simulink library "IOBlock_Library_TTC580"  (R2021a)
settings: Solver=ode45  StartTime=0.0  StopTime=10.0  RelTol=1e-3
PreLoadFcn:
  | addpath(genpath(fileparts(which('IOBlock_Library_TTC580'))));
  | %addpath(genpath(fileparts(which('IOBlock_Library_TTC580.mdl'))))
  | try
  | addpath(genpath([fileparts(which('IOBlock_Library_TTC580')),'\..\DBC_Importer']));
  | addpath(genpath([fileparts(which('IOBlock_Library_TTC580')),'\..\EEPROM_Importer']));
  | addpath(genpath([fileparts(which('IOBlock_Library_TTC580')),'\..\UserDoc']));
  | catch
  | warning('IOBlock_Library_TTC580: add path to DBC_Importer and EEPROM_Importer manually');
  | end
  | try
  | if exist('..\CustomPackage\scripts\OpenAllPackages.m','file')
  |      run('..\CustomPackage\scripts\OpenAllPackages.m'); %always available, ggf. empty
  | end
  | catch
  | warning('A problem occurred opening automatically the CustomPackage. Please open libraries manually');
  | end
  | try
  | set_param(0,'EditorSmartEditingHotParam','off');
  | catch
  | warning('Simlink preferences for ''Edit key parameter when adding new blocks'' needs to be unchecked manually');
  | end
undefined symbols (not defined in the file or in its folder): ADC_Absolute_10V, ADC_Absolute_32V, ADC_Absolute_5V, ADC_BoardTemp, ADC_ChannelInit, ADC_Current, ADC_Get, ADC_K15_, ADC_Ratiometric_10V, ADC_Ratiometric_5V, ADC_Resistive, ADC_SensorSupply, ADC_UBAT, bit_packing, bit_unpacking, CAN_ConfigMsg, compare2error, compare2FET_PROT_REENABLE, crc32_calc_intern, CRC32_EEPROM_Read, CRC32_EEPROM_Write, DIAG_EnterSafestate, DIAG_Status, DIAG_Status_internal, EEPROM_Mirror, EEPROM_Read, EEPROM_Read_OffsetIn, EEPROM_Read_Raw, EEPROM_Write, EEPROM_Write_OffsetIn, EEPROM_Write_Raw, EnterSafestate, FPU_Handler, Get_DI, Get_DI_VarThreshold, Get_K15_, Get_Pulse_Freq_Curr, Get_Pulse_Freq_Volt, Get_WakeUp, GetDateAndTime, IO_ADC_ResetProtection, IO_Blk_Lib_TTC500, IO_CAN_ReadMsg, IO_CAN_WriteMsg, IO_DI_Get, IO_DI_Init, IO_DI_Init_Var, IO_DO_GetCur, IO_DO_GetVoltage, IO_DO_Init, IO_DO_ResetProtection, IO_DO_Set, IO_Driver_GetSerialNumber, IO_Driver_GetVersionOfDriver, IO_Driver_GetVersionOfFPGA, IO_EEPROM_GetStatus, IO_EEPROM_Init, IO_EEPROM_Read_raw, IO_EEPROM_Write, IO_EEPROM_Write_OffsetIn ... (+73)
libraries: simulink x43
(part 14 of 18)

== system IOBlock_Library_TTC580/PWM Blocks TTC580 IOlib/Set_PWM_Simple ==
  duty_cycle : Inport  OutDataTypeStr=uint16  PortDimensions=1
  IO_PWM_Init : Subsystem  LoadFcn=|  mask(IO_PWM_Init_Code){SampleTime=-1, ttlib=IO_Blk_Lib_TTC500, ttDescription=IO_PWM_Init, tt_iolib_version=0.19, pwm_channel=pwm_channel, frequency=frequency, polarity=num2str(polarity_high), diag_margin=num2str(diag_margin), safety_conf=NULL}
      | try
      | %
      | %Upgrade Information - standard BEGIN
      | new_color = 'blue';
      | new_ver = '0.19';
      | act_ver = get_param(gcb,'tt_iolib_version');
      | if not(strcmp(act_ver,new_ver))
      |     disp(['Upgrade block: ',gcb,char(10),'       Version: ',act_ver,' -> ',new_ver]);
      |     %switch - case for specific upgrade information e.g. additional parameter required 
      |     %Change appearance and version information
      |     set_param(gcb,'ForegroundColor',new_color);
      |     set_param(gcb,'tt_iolib_version',new_ver);
      | end
      | %Upgrade Information - standard END
      | catch
      | %Standard catch section BEGIN 
      | disp(' ');
      | disp('------------------------------------------------------------');
      | disp('An error occurred in a callback of the TTC580-BlockLib.');
      | disp(['Please check the parameters in the mask of ',gcb]);
      | disp('If you do not encounter any violations, then please '); 
      | disp('copy the following lines and report this to support@ttcontrol.com ');
      | disp('<< begin of error message dump >>');
      | disp(['Version of TTC580-BlockLib: ', get_param(gcb,'tt_iolib_version')]);
      | disp(get_param(gcb,'ttDescription'));
      | disp(gcb);
      | x=lasterror;disp(x.message);
      | disp(get_param(gcb,'MaskValues'));
      | disp(version);
      | disp(computer);
      | disp('<< end of error message dump >>');
      | disp('------------------------------------------------------------');
      | disp(' ');
      | %Standard catch section END
      | end
      mask help: Setup single PWM output.
      mask init:
      | %
      settings: CopyFcn=%deleted
      mask Help: web(which('IO_PWM.h'))
      mask Callback pwm_channel: %
      mask Callback frequency: %
      mask Callback polarity: %
      mask Callback diag_margin: %
      mask Callback safety_conf: %
  IO_PWM_ResetProtection : Subsystem  LoadFcn=|  mask(IO_PWM_ResetProtection_Code){SampleTime=-1, ttlib=IO_Blk_Lib_TTC500, ttDescription=IO_PWM_ResetProtection, tt_iolib_version=0.19, pwm_channel=pwm_channel}
      | try
      | %
      | %Upgrade Information - standard BEGIN
      | new_color = 'blue';
      | new_ver = '0.19';
      | act_ver = get_param(gcb,'tt_iolib_version');
      | if not(strcmp(act_ver,new_ver))
      |     disp(['Upgrade block: ',gcb,char(10),'       Version: ',act_ver,' -> ',new_ver]);
      |     %switch - case for specific upgrade information e.g. additional parameter required 
      |     %Change appearance and version information
      |     set_param(gcb,'ForegroundColor',new_color);
      |     set_param(gcb,'tt_iolib_version',new_ver);
      | end
      | %Upgrade Information - standard END
      | catch
      | %Standard catch section BEGIN 
      | disp(' ');
      | disp('------------------------------------------------------------');
      | disp('An error occurred in a callback of the TTC580-BlockLib.');
      | disp(['Please check the parameters in the mask of ',gcb]);
      | disp('If you do not encounter any violations, then please '); 
      | disp('copy the following lines and report this to support@ttcontrol.com ');
      | disp('<< begin of error message dump >>');
      | disp(['Version of TTC580-BlockLib: ', get_param(gcb,'tt_iolib_version')]);
      | disp(get_param(gcb,'ttDescription'));
      | disp(gcb);
      | x=lasterror;disp(x.message);
      | disp(get_param(gcb,'MaskValues'));
      | disp(version);
      | disp(computer);
      | disp('<< end of error message dump >>');
      | disp('------------------------------------------------------------');
      | disp(' ');
      | %Standard catch section END
      | end
      mask help: Reset the output protection for a PWM channel.
      mask init:
      | %
      settings: CopyFcn=%deleted
      mask Help: web(which('IO_PWM.h'))
      mask Callback pwm_channel: %
  PWM_Init : Terminator
  PWM_SetDuty_Simple : Subsystem  LoadFcn=|  mask(PWM_SetDuty_Simple_Code){SampleTime=-1, ttlib=IO_Blk_Lib_TTC500, ttDescription=PWM_SetDuty_Simple, tt_iolib_version=0.19, pwm_channel=pwm_channel, high_time_fb=NULL, period_fb=NULL}
      | try
      | %
      | %Upgrade Information - standard BEGIN
      | new_color = 'blue';
      | new_ver = '0.19';
      | act_ver = get_param(gcb,'tt_iolib_version');
      | if not(strcmp(act_ver,new_ver))
      |     disp(['Upgrade block: ',gcb,char(10),'       Version: ',act_ver,' -> ',new_ver]);
      |     %switch - case for specific upgrade information e.g. additional parameter required 
      |     %Change appearance and version information
      |     set_param(gcb,'ForegroundColor',new_color);
      |     set_param(gcb,'tt_iolib_version',new_ver);
      | end
      | %Upgrade Information - standard END
      | catch
      | %Standard catch section BEGIN 
      | disp(' ');
      | disp('------------------------------------------------------------');
      | disp('An error occurred in a callback of the TTC580-BlockLib.');
      | disp(['Please check the parameters in the mask of ',gcb]);
      | disp('If you do not encounter any violations, then please '); 
      | disp('copy the following lines and report this to support@ttcontrol.com ');
      | disp('<< begin of error message dump >>');
      | disp(['Version of TTC580-BlockLib: ', get_param(gcb,'tt_iolib_version')]);
      | disp(get_param(gcb,'ttDescription'));
      | disp(gcb);
      | x=lasterror;disp(x.message);
      | disp(get_param(gcb,'MaskValues'));
      | disp(version);
      | disp(computer);
      | disp('<< end of error message dump >>');
      | disp('------------------------------------------------------------');
      | disp(' ');
      | %Standard catch section END
      | end
      mask help: Set the duty cycle for a PWM channel.
      mask init:
      | %
      settings: CopyFcn=%deleted
      mask Help: web(which('IO_PWM.h'))
      mask Callback pwm_channel: %
      mask Callback high_time_fb: %
      mask Callback period_fb: %
  Terminator1 : Terminator
  Terminator3 : Terminator
  compare2FET_PROT_REENABLE : Subsystem  LoadFcn=|  mask(compare2FET_PROT_REENABLE_Code){SampleTime=-1, ttlib=IO_Blk_Lib_TTC500, ttDescription=compare2FET_PROT_REENABLE, tt_iolib_version=0.19, define=IO_E_FET_PROT_REENABLE}
      | try
      | %
      | %Upgrade Information - standard BEGIN
      | new_color = 'blue';
      | new_ver = '0.19';
      | act_ver = get_param(gcb,'tt_iolib_version');
      | if not(strcmp(act_ver,new_ver))
      |     disp(['Upgrade block: ',gcb,char(10),'       Version: ',act_ver,' -> ',new_ver]);
      |     %switch - case for specific upgrade information e.g. additional parameter required 
      |     %Change appearance and version information
      |     set_param(gcb,'ForegroundColor',new_color);
      |     set_param(gcb,'tt_iolib_version',new_ver);
      | end
      | %Upgrade Information - standard END
      | catch
      | %Standard catch section BEGIN 
      | disp(' ');
      | disp('------------------------------------------------------------');
      | disp('An error occurred in a callback of the TTC580-BlockLib.');
      | disp(['Please check the parameters in the mask of ',gcb]);
      | disp('If you do not encounter any violations, then please '); 
      | disp('copy the following lines and report this to support@ttcontrol.com ');
      | disp('<< begin of error message dump >>');
      | disp(['Version of TTC580-BlockLib: ', get_param(gcb,'tt_iolib_version')]);
      | disp(get_param(gcb,'ttDescription'));
      | disp(gcb);
      | x=lasterror;disp(x.message);
      | disp(get_param(gcb,'MaskValues'));
      | disp(version);
      | disp(computer);
      | disp('<< end of error message dump >>');
      | disp('------------------------------------------------------------');
      | disp(' ');
      | %Standard catch section END
      | end
      mask help: The ErrorCode that is output from an I/O-Block is compared against IO_E_FET_PROT_REENABLE.
      mask init:
      | %
      settings: CopyFcn=%deleted
      mask Help: web(which('~.h'))
      mask Callback define: %
  ErrorCode : Outport  VectorParamsAs1DForOutWhenUnconnected=off
  wires:
  IO_PWM_Init/1(ErrorCode) -> PWM_Init/1
  duty_cycle/1 -> PWM_SetDuty_Simple/1(duty_cycle)
  PWM_SetDuty_Simple/1(ErrorCode) -> ErrorCode/1, compare2FET_PROT_REENABLE/1(Errorcode)
  compare2FET_PROT_REENABLE/1(b_compare) -> IO_PWM_ResetProtection/Trigger
  IO_PWM_ResetProtection/1(ErrorCode) -> Terminator3/1
  IO_PWM_ResetProtection/2(reset_cnt) -> Terminator1/1

== system IOBlock_Library_TTC580/SensorSupply TTC580 IOlib/SensorSupply_5V ==
  enable : Inport  OutDataTypeStr=boolean  PortDimensions=1
  Data Type Conversion : DataTypeConversion  OutDataTypeStr=uint8
  POWER_Set_Output : Subsystem  LoadFcn=|  mask(POWER_Set_Output_Code){SampleTime=-1, ttlib=IO_Blk_Lib_TTC500, ttDescription=POWER_Set_Output, tt_iolib_version=0.19, pin=sensor_supply}
      | try
      | %
      | %Upgrade Information - standard BEGIN
      | new_color = 'blue';
      | new_ver = '0.19';
      | act_ver = get_param(gcb,'tt_iolib_version');
      | if not(strcmp(act_ver,new_ver))
      |     disp(['Upgrade block: ',gcb,char(10),'       Version: ',act_ver,' -> ',new_ver]);
      |     %switch - case for specific upgrade information e.g. additional parameter required 
      |     %Change appearance and version information
      |     set_param(gcb,'ForegroundColor',new_color);
      |     set_param(gcb,'tt_iolib_version',new_ver);
      | end
      | %Upgrade Information - standard END
      | catch
      | %Standard catch section BEGIN 
      | disp(' ');
      | disp('------------------------------------------------------------');
      | disp('An error occurred in a callback of the TTC580-BlockLib.');
      | disp(['Please check the parameters in the mask of ',gcb]);
      | disp('If you do not encounter any violations, then please '); 
      | disp('copy the following lines and report this to support@ttcontrol.com ');
      | disp('<< begin of error message dump >>');
      | disp(['Version of TTC580-BlockLib: ', get_param(gcb,'tt_iolib_version')]);
      | disp(get_param(gcb,'ttDescription'));
      | disp(gcb);
      | x=lasterror;disp(x.message);
      | disp(get_param(gcb,'MaskValues'));
      | disp(version);
      | disp(computer);
      | disp('<< end of error message dump >>');
      | disp('------------------------------------------------------------');
      | disp(' ');
      | %Standard catch section END
      | end
      mask help: Sets a certain mode of the Power IC.
      mask init:
      | %
      settings: CopyFcn=%deleted
      mask Help: No further help available for this block
      mask Callback pin: %
  ErrorCode : Outport  VectorParamsAs1DForOutWhenUnconnected=off
  wires:
  enable/1 -> Data Type Conversion/1
  POWER_Set_Output/1(ErrorCode) -> ErrorCode/1
  Data Type Conversion/1 -> POWER_Set_Output/1(mode)

== system IOBlock_Library_TTC580/SensorSupply TTC580 IOlib/SensorSupply_Modif ==
  Volt : Inport  OutDataTypeStr=uint8  PortDimensions=1
  POWER_Set_Output : Subsystem  LoadFcn=|  mask(POWER_Set_Output_Code){SampleTime=-1, ttlib=IO_Blk_Lib_TTC500, ttDescription=POWER_Set_Output, tt_iolib_version=0.19, pin=sensor_supply}
      | try
      | %
      | %Upgrade Information - standard BEGIN
      | new_color = 'blue';
      | new_ver = '0.19';
      | act_ver = get_param(gcb,'tt_iolib_version');
      | if not(strcmp(act_ver,new_ver))
      |     disp(['Upgrade block: ',gcb,char(10),'       Version: ',act_ver,' -> ',new_ver]);
      |     %switch - case for specific upgrade information e.g. additional parameter required 
      |     %Change appearance and version information
      |     set_param(gcb,'ForegroundColor',new_color);
      |     set_param(gcb,'tt_iolib_version',new_ver);
      | end
      | %Upgrade Information - standard END
      | catch
      | %Standard catch section BEGIN 
      | disp(' ');
      | disp('------------------------------------------------------------');
      | disp('An error occurred in a callback of the TTC580-BlockLib.');
      | disp(['Please check the parameters in the mask of ',gcb]);
      | disp('If you do not encounter any violations, then please '); 
      | disp('copy the following lines and report this to support@ttcontrol.com ');
      | disp('<< begin of error message dump >>');
      | disp(['Version of TTC580-BlockLib: ', get_param(gcb,'tt_iolib_version')]);
      | disp(get_param(gcb,'ttDescription'));
      | disp(gcb);
      | x=lasterror;disp(x.message);
      | disp(get_param(gcb,'MaskValues'));
      | disp(version);
      | disp(computer);
      | disp('<< end of error message dump >>');
      | disp('------------------------------------------------------------');
      | disp(' ');
      | %Standard catch section END
      | end
      mask help: Sets a certain mode of the Power IC.
      mask init:
      | %
      settings: CopyFcn=%deleted
      mask Help: No further help available for this block
      mask Callback pin: %
  Volt_to_mode : LookupNDDirect  NumberOfTableDimensions=1  Table=uint8([0 0 0 0 0 2 3 4 5 6 7 0])  DiagnosticForOutOfRangeInput=None
  ErrorCode : Outport  VectorParamsAs1DForOutWhenUnconnected=off
  wires:
  POWER_Set_Output/1(ErrorCode) -> ErrorCode/1
  Volt/1 -> Volt_to_mode/1
  Volt_to_mode/1 -> POWER_Set_Output/1(mode)

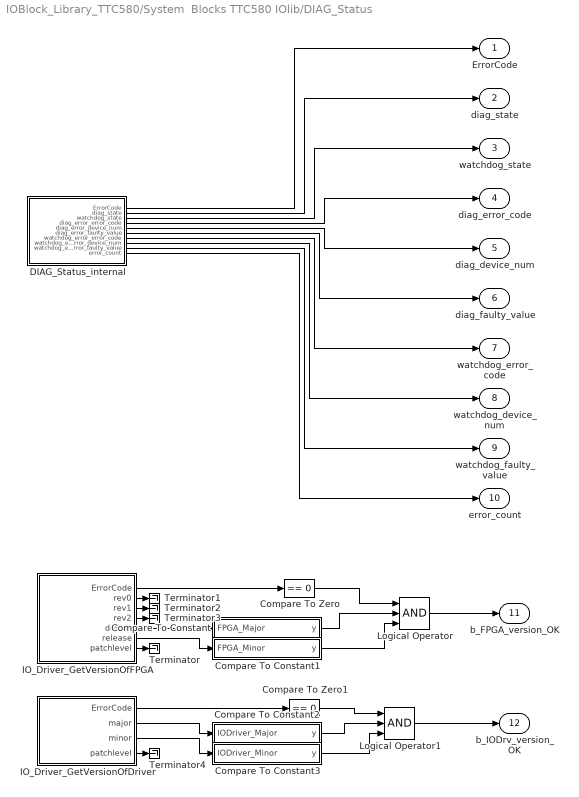
== system IOBlock_Library_TTC580/System  Blocks TTC580 IOlib/DIAG_Status ==
  Compare To Constant : Subsystem
  Compare To Constant1 : Subsystem
  Compare To Constant2 : Subsystem
  Compare To Constant3 : Subsystem
  Compare To Zero : simulink/Logic and Bit Operations/Compare To Zero  relop===  OutDataTypeStr=boolean  ZeroCross=off
  Compare To Zero1 : simulink/Logic and Bit Operations/Compare To Zero  relop===  OutDataTypeStr=boolean  ZeroCross=off
  DIAG_Status_internal : Subsystem  LoadFcn=|  mask(DIAG_Status_internal_Code){SampleTime=-1, ttlib=IO_Blk_Lib_TTC500, ttDescription=DIAG_Status_internal, tt_iolib_version=0.19}
      | try
      | %
      | %Upgrade Information - standard BEGIN
      | new_color = 'blue';
      | new_ver = '0.19';
      | act_ver = get_param(gcb,'tt_iolib_version');
      | if not(strcmp(act_ver,new_ver))
      |     disp(['Upgrade block: ',gcb,char(10),'       Version: ',act_ver,' -> ',new_ver]);
      |     %switch - case for specific upgrade information e.g. additional parameter required 
      |     %Change appearance and version information
      |     set_param(gcb,'ForegroundColor',new_color);
      |     set_param(gcb,'tt_iolib_version',new_ver);
      | end
      | %Upgrade Information - standard END
      | catch
      | %Standard catch section BEGIN 
      | disp(' ');
      | disp('------------------------------------------------------------');
      | disp('An error occurred in a callback of the TTC580-BlockLib.');
      | disp(['Please check the parameters in the mask of ',gcb]);
      | disp('If you do not encounter any violations, then please '); 
      | disp('copy the following lines and report this to support@ttcontrol.com ');
      | disp('<< begin of error message dump >>');
      | disp(['Version of TTC580-BlockLib: ', get_param(gcb,'tt_iolib_version')]);
      | disp(get_param(gcb,'ttDescription'));
      | disp(gcb);
      | x=lasterror;disp(x.message);
      | disp(get_param(gcb,'MaskValues'));
      | disp(version);
      | disp(computer);
      | disp('<< end of error message dump >>');
      | disp('------------------------------------------------------------');
      | disp(' ');
      | %Standard catch section END
      | end
      mask help: Status function for diagnostic state machine and watchdog states.
      mask init:
      | %
      settings: CopyFcn=%deleted
      mask Help: web(which('DIAG_Functions.h'))
  IO_Driver_GetVersionOfDriver : Subsystem  LoadFcn=|  mask(IO_Driver_GetVersionOfDriver_Code){SampleTime=-1, ttlib=IO_Blk_Lib_TTC500, ttDescription=IO_Driver_GetVersionOfDriver, tt_iolib_version=0.19}
      | try
      | %
      | %Upgrade Information - standard BEGIN
      | new_color = 'blue';
      | new_ver = '0.19';
      | act_ver = get_param(gcb,'tt_iolib_version');
      | if not(strcmp(act_ver,new_ver))
      |     disp(['Upgrade block: ',gcb,char(10),'       Version: ',act_ver,' -> ',new_ver]);
      |     %switch - case for specific upgrade information e.g. additional parameter required 
      |     %Change appearance and version information
      |     set_param(gcb,'ForegroundColor',new_color);
      |     set_param(gcb,'tt_iolib_version',new_ver);
      | end
      | %Upgrade Information - standard END
      | catch
      | %Standard catch section BEGIN 
      | disp(' ');
      | disp('------------------------------------------------------------');
      | disp('An error occurred in a callback of the TTC580-BlockLib.');
      | disp(['Please check the parameters in the mask of ',gcb]);
      | disp('If you do not encounter any violations, then please '); 
      | disp('copy the following lines and report this to support@ttcontrol.com ');
      | disp('<< begin of error message dump >>');
      | disp(['Version of TTC580-BlockLib: ', get_param(gcb,'tt_iolib_version')]);
      | disp(get_param(gcb,'ttDescription'));
      | disp(gcb);
      | x=lasterror;disp(x.message);
      | disp(get_param(gcb,'MaskValues'));
      | disp(version);
      | disp(computer);
      | disp('<< end of error message dump >>');
      | disp('------------------------------------------------------------');
      | disp(' ');
      | %Standard catch section END
      | end
      mask help: Returns the version number of the IO driver.
      mask init:
      | %
      settings: CopyFcn=%deleted
      mask Help: web(which('IO_Driver.h'))
  IO_Driver_GetVersionOfFPGA : Subsystem  LoadFcn=|  mask(IO_Driver_GetVersionOfFPGA_Code){SampleTime=-1, ttlib=IO_Blk_Lib_TTC500, ttDescription=IO_Driver_GetVersionOfFPGA, tt_iolib_version=0.19}
      | try
      | %
      | %Upgrade Information - standard BEGIN
      | new_color = 'blue';
      | new_ver = '0.19';
      | act_ver = get_param(gcb,'tt_iolib_version');
      | if not(strcmp(act_ver,new_ver))
      |     disp(['Upgrade block: ',gcb,char(10),'       Version: ',act_ver,' -> ',new_ver]);
      |     %switch - case for specific upgrade information e.g. additional parameter required 
      |     %Change appearance and version information
      |     set_param(gcb,'ForegroundColor',new_color);
      |     set_param(gcb,'tt_iolib_version',new_ver);
      | end
      | %Upgrade Information - standard END
      | catch
      | %Standard catch section BEGIN 
      | disp(' ');
      | disp('------------------------------------------------------------');
      | disp('An error occurred in a callback of the TTC580-BlockLib.');
      | disp(['Please check the parameters in the mask of ',gcb]);
      | disp('If you do not encounter any violations, then please '); 
      | disp('copy the following lines and report this to support@ttcontrol.com ');
      | disp('<< begin of error message dump >>');
      | disp(['Version of TTC580-BlockLib: ', get_param(gcb,'tt_iolib_version')]);
      | disp(get_param(gcb,'ttDescription'));
      | disp(gcb);
      | x=lasterror;disp(x.message);
      | disp(get_param(gcb,'MaskValues'));
      | disp(version);
      | disp(computer);
      | disp('<< end of error message dump >>');
      | disp('------------------------------------------------------------');
      | disp(' ');
      | %Standard catch section END
      | end
      mask help: Returns the version number of the FPGA IP.
      mask init:
      | %
      settings: CopyFcn=%deleted
      mask Help: web(which('IO_Driver.h'))
  Logical Operator : Logic  Inputs=3  AllPortsSameDT=off  OutDataTypeStr=boolean
  Logical Operator1 : Logic  Inputs=3  AllPortsSameDT=off  OutDataTypeStr=boolean
  Terminator{,1..4} (5 alike) : Terminator
  ErrorCode : Outport  VectorParamsAs1DForOutWhenUnconnected=off
  diag_state : Outport  Port=2  VectorParamsAs1DForOutWhenUnconnected=off
  watchdog_state : Outport  Port=3  VectorParamsAs1DForOutWhenUnconnected=off
  diag_error_code : Outport  Port=4  VectorParamsAs1DForOutWhenUnconnected=off
  diag_device_num : Outport  Port=5  VectorParamsAs1DForOutWhenUnconnected=off
  diag_faulty_value : Outport  Port=6  VectorParamsAs1DForOutWhenUnconnected=off
  watchdog_error_code : Outport  Port=7  VectorParamsAs1DForOutWhenUnconnected=off
  watchdog_device_num : Outport  Port=8  VectorParamsAs1DForOutWhenUnconnected=off
  watchdog_faulty_value : Outport  Port=9  VectorParamsAs1DForOutWhenUnconnected=off
  error_count : Outport  Port=10  VectorParamsAs1DForOutWhenUnconnected=off
  b_FPGA_version_OK : Outport  Port=11  VectorParamsAs1DForOutWhenUnconnected=off
  b_IODrv_version_OK : Outport  Port=12  VectorParamsAs1DForOutWhenUnconnected=off
  wires:
  Compare To Constant3/1(y) -> Logical Operator1/3
  Compare To Constant2/1(y) -> Logical Operator1/2
  Compare To Constant1/1(y) -> Logical Operator/3
  Compare To Constant/1(y) -> Logical Operator/2
  Logical Operator1/1 -> b_IODrv_version_OK/1
  Compare To Zero1/1 -> Logical Operator1/1
  Logical Operator/1 -> b_FPGA_version_OK/1
  Compare To Zero/1 -> Logical Operator/1
  IO_Driver_GetVersionOfDriver/1(ErrorCode) -> Compare To Zero1/1
  IO_Driver_GetVersionOfFPGA/1(ErrorCode) -> Compare To Zero/1
  IO_Driver_GetVersionOfDriver/4(patchlevel) -> Terminator4/1
  IO_Driver_GetVersionOfFPGA/4(rev2) -> Terminator3/1
  IO_Driver_GetVersionOfFPGA/3(rev1) -> Terminator2/1
  IO_Driver_GetVersionOfFPGA/2(rev0) -> Terminator1/1
  IO_Driver_GetVersionOfFPGA/7(patchlevel) -> Terminator/1
  IO_Driver_GetVersionOfDriver/3(minor) -> Compare To Constant3/1(IODriver_Minor)
  IO_Driver_GetVersionOfDriver/2(major) -> Compare To Constant2/1(IODriver_Major)
  IO_Driver_GetVersionOfFPGA/6(release) -> Compare To Constant1/1(FPGA_Minor)
  IO_Driver_GetVersionOfFPGA/5(device) -> Compare To Constant/1(FPGA_Major)
  DIAG_Status_internal/10(error_count) -> error_count/1
  DIAG_Status_internal/9(watchdog_error_faulty_value) -> watchdog_faulty_value/1
  DIAG_Status_internal/8(watchdog_error_device_num) -> watchdog_device_num/1
  DIAG_Status_internal/7(watchdog_error_error_code) -> watchdog_error_code/1
  DIAG_Status_internal/6(diag_error_faulty_value) -> diag_faulty_value/1
  DIAG_Status_internal/5(diag_error_device_num) -> diag_device_num/1
  DIAG_Status_internal/4(diag_error_error_code) -> diag_error_code/1
  DIAG_Status_internal/3(watchdog_state) -> watchdog_state/1
  DIAG_Status_internal/2(diag_state) -> diag_state/1
  DIAG_Status_internal/1(ErrorCode) -> ErrorCode/1

== system IOBlock_Library_TTC580/System  Blocks TTC580 IOlib/EnterSafestate ==
  enable : Inport  OutDataTypeStr=boolean  PortDimensions=1
  DIAG_EnterSafestate_x : Subsystem  LoadFcn=|  mask(DIAG_EnterSafestate_Code){SampleTime=-1, ttlib=IO_Blk_Lib_TTC500, ttDescription=DIAG_EnterSafestate, tt_iolib_version=0.19}
      | try
      | %
      | %Upgrade Information - standard BEGIN
      | new_color = 'blue';
      | new_ver = '0.19';
      | act_ver = get_param(gcb,'tt_iolib_version');
      | if not(strcmp(act_ver,new_ver))
      |     disp(['Upgrade block: ',gcb,char(10),'       Version: ',act_ver,' -> ',new_ver]);
      |     %switch - case for specific upgrade information e.g. additional parameter required 
      |     %Change appearance and version information
      |     set_param(gcb,'ForegroundColor',new_color);
      |     set_param(gcb,'tt_iolib_version',new_ver);
      | end
      | %Upgrade Information - standard END
      | catch
      | %Standard catch section BEGIN 
      | disp(' ');
      | disp('------------------------------------------------------------');
      | disp('An error occurred in a callback of the TTC580-BlockLib.');
      | disp(['Please check the parameters in the mask of ',gcb]);
      | disp('If you do not encounter any violations, then please '); 
      | disp('copy the following lines and report this to support@ttcontrol.com ');
      | disp('<< begin of error message dump >>');
      | disp(['Version of TTC580-BlockLib: ', get_param(gcb,'tt_iolib_version')]);
      | disp(get_param(gcb,'ttDescription'));
      | disp(gcb);
      | x=lasterror;disp(x.message);
      | disp(get_param(gcb,'MaskValues'));
      | disp(version);
      | disp(computer);
      | disp('<< end of error message dump >>');
      | disp('------------------------------------------------------------');
      | disp(' ');
      | %Standard catch section END
      | end
      mask help: Allows an application driven safe state.
      mask init:
      | %
      settings: CopyFcn=%deleted
      mask Help: web(which('DIAG_Functions.h'))
  Terminator_enabe : Terminator
  wires:
  DIAG_EnterSafestate_x/1(ErrorCode) -> Terminator_enabe/1
  enable/1 -> DIAG_EnterSafestate_x/Enable

== system IOBlock_Library_TTC580/System  Blocks TTC580 IOlib/FPU_Handler ==
  FPU_Handler_s : S-Function  FunctionName=FPU_Handler_s  Parameters=SampleTime,division_by_zero,input_denormal,invalid_operation,overflow,underflow  SFunctionDeploymentMode=off  EnableBusSupport=off

== system IOBlock_Library_TTC580/System  Blocks TTC580 IOlib/GetDateAndTime ==
  trigger : Inport  OutDataTypeStr=boolean  PortDimensions=1
  IO_RTC_GetDateAndTime : Subsystem  LoadFcn=|  mask(IO_RTC_GetDateAndTime_Code){SampleTime=-1, ttlib=IO_Blk_Lib_TTC500, ttDescription=IO_RTC_GetDateAndTime, tt_iolib_version=0.19}
      | try
      | %
      | %Upgrade Information - standard BEGIN
      | new_color = 'blue';
      | new_ver = '0.19';
      | act_ver = get_param(gcb,'tt_iolib_version');
      | if not(strcmp(act_ver,new_ver))
      |     disp(['Upgrade block: ',gcb,char(10),'       Version: ',act_ver,' -> ',new_ver]);
      |     %switch - case for specific upgrade information e.g. additional parameter required 
      |     %Change appearance and version information
      |     set_param(gcb,'ForegroundColor',new_color);
      |     set_param(gcb,'tt_iolib_version',new_ver);
      | end
      | %Upgrade Information - standard END
      | catch
      | %Standard catch section BEGIN 
      | disp(' ');
      | disp('------------------------------------------------------------');
      | disp('An error occurred in a callback of the TTC580-BlockLib.');
      | disp(['Please check the parameters in the mask of ',gcb]);
      | disp('If you do not encounter any violations, then please '); 
      | disp('copy the following lines and report this to support@ttcontrol.com ');
      | disp('<< begin of error message dump >>');
      | disp(['Version of TTC580-BlockLib: ', get_param(gcb,'tt_iolib_version')]);
      | disp(get_param(gcb,'ttDescription'));
      | disp(gcb);
      | x=lasterror;disp(x.message);
      | disp(get_param(gcb,'MaskValues'));
      | disp(version);
      | disp(computer);
      | disp('<< end of error message dump >>');
      | disp('------------------------------------------------------------');
      | disp(' ');
      | %Standard catch section END
      | end
      mask help: Returns the date and time of the real time clock.
      mask init:
      | %
      settings: CopyFcn=%deleted
      mask Help: No further help available for this block
  IO_RTC_GetDateAndTimeStatus : Subsystem  LoadFcn=|  mask(IO_RTC_GetDateAndTimeStatus_Code){SampleTime=-1, ttlib=IO_Blk_Lib_TTC500, ttDescription=IO_RTC_GetDateAndTimeStatus, tt_iolib_version=0.19}
      | try
      | %
      | %Upgrade Information - standard BEGIN
      | new_color = 'blue';
      | new_ver = '0.19';
      | act_ver = get_param(gcb,'tt_iolib_version');
      | if not(strcmp(act_ver,new_ver))
      |     disp(['Upgrade block: ',gcb,char(10),'       Version: ',act_ver,' -> ',new_ver]);
      |     %switch - case for specific upgrade information e.g. additional parameter required 
      |     %Change appearance and version information
      |     set_param(gcb,'ForegroundColor',new_color);
      |     set_param(gcb,'tt_iolib_version',new_ver);
      | end
      | %Upgrade Information - standard END
      | catch
      | %Standard catch section BEGIN 
      | disp(' ');
      | disp('------------------------------------------------------------');
      | disp('An error occurred in a callback of the TTC580-BlockLib.');
      | disp(['Please check the parameters in the mask of ',gcb]);
      | disp('If you do not encounter any violations, then please '); 
      | disp('copy the following lines and report this to support@ttcontrol.com ');
      | disp('<< begin of error message dump >>');
      | disp(['Version of TTC580-BlockLib: ', get_param(gcb,'tt_iolib_version')]);
      | disp(get_param(gcb,'ttDescription'));
      | disp(gcb);
      | x=lasterror;disp(x.message);
      | disp(get_param(gcb,'MaskValues'));
      | disp(version);
      | disp(computer);
      | disp('<< end of error message dump >>');
      | disp('------------------------------------------------------------');
      | disp(' ');
      | %Standard catch section END
      | end
      mask help: Gets the status of the external RTC device.
      mask init:
      | %
      settings: CopyFcn=%deleted
      mask Help: No further help available for this block
  IO_RTC_InitDateAndTime : Subsystem  LoadFcn=|  mask(IO_RTC_InitDateAndTime_Code){SampleTime=-1, ttlib=IO_Blk_Lib_TTC500, ttDescription=IO_RTC_InitDateAndTime, tt_iolib_version=0.19}
      | try
      | %
      | %Upgrade Information - standard BEGIN
      | new_color = 'blue';
      | new_ver = '0.19';
      | act_ver = get_param(gcb,'tt_iolib_version');
      | if not(strcmp(act_ver,new_ver))
      |     disp(['Upgrade block: ',gcb,char(10),'       Version: ',act_ver,' -> ',new_ver]);
      |     %switch - case for specific upgrade information e.g. additional parameter required 
      |     %Change appearance and version information
      |     set_param(gcb,'ForegroundColor',new_color);
      |     set_param(gcb,'tt_iolib_version',new_ver);
      | end
      | %Upgrade Information - standard END
      | catch
      | %Standard catch section BEGIN 
      | disp(' ');
      | disp('------------------------------------------------------------');
      | disp('An error occurred in a callback of the TTC580-BlockLib.');
      | disp(['Please check the parameters in the mask of ',gcb]);
      | disp('If you do not encounter any violations, then please '); 
      | disp('copy the following lines and report this to support@ttcontrol.com ');
      | disp('<< begin of error message dump >>');
      | disp(['Version of TTC580-BlockLib: ', get_param(gcb,'tt_iolib_version')]);
      | disp(get_param(gcb,'ttDescription'));
      | disp(gcb);
      | x=lasterror;disp(x.message);
      | disp(get_param(gcb,'MaskValues'));
      | disp(version);
      | disp(computer);
      | disp('<< end of error message dump >>');
      | disp('------------------------------------------------------------');
      | disp(' ');
      | %Standard catch section END
      | end
      mask help: Initializes the external RTC device for date and time operations.
      mask init:
      | %
      settings: CopyFcn=%deleted
      mask Help: No further help available for this block
  Terminator : Terminator
  Status : Outport  VectorParamsAs1DForOutWhenUnconnected=off
  seconds : Outport  Port=2  VectorParamsAs1DForOutWhenUnconnected=off
  minutes : Outport  Port=3  VectorParamsAs1DForOutWhenUnconnected=off
  hours : Outport  Port=4  VectorParamsAs1DForOutWhenUnconnected=off
  days : Outport  Port=5  VectorParamsAs1DForOutWhenUnconnected=off
  months : Outport  Port=6  VectorParamsAs1DForOutWhenUnconnected=off
  years : Outport  Port=7  VectorParamsAs1DForOutWhenUnconnected=off
  wires:
  IO_RTC_GetDateAndTime/7(years) -> years/1
  IO_RTC_GetDateAndTime/6(months) -> months/1
  IO_RTC_GetDateAndTime/5(days) -> days/1
  IO_RTC_GetDateAndTime/4(hours) -> hours/1
  IO_RTC_GetDateAndTime/3(minutes) -> minutes/1
  IO_RTC_GetDateAndTime/2(seconds) -> seconds/1
  IO_RTC_GetDateAndTimeStatus/1(ErrorCode) -> Status/1
  IO_RTC_GetDateAndTime/1(ErrorCode) -> IO_RTC_GetDateAndTimeStatus/1(logical_link)
  IO_RTC_InitDateAndTime/1(ErrorCode) -> Terminator/1
  trigger/1 -> IO_RTC_GetDateAndTime/Trigger

== system IOBlock_Library_TTC580/System  Blocks TTC580 IOlib/IO_Driver_GetSerialNumber ==
  IO_Driver_GetSerialNumber_s : S-Function  FunctionName=IO_Driver_GetSerialNumber_s  Parameters=SampleTime  SFunctionDeploymentMode=off  EnableBusSupport=off
  ErrorCode : Outport  VectorParamsAs1DForOutWhenUnconnected=off
  serialnumber : Outport  Port=2  VectorParamsAs1DForOutWhenUnconnected=off
  wires:
  IO_Driver_GetSerialNumber_s/2 -> serialnumber/1
  IO_Driver_GetSerialNumber_s/1 -> ErrorCode/1

== system IOBlock_Library_TTC580/System  Blocks TTC580 IOlib/MainDlg ==
  MainDlg_basic : Subsystem  Priority=-2147483646  LoadFcn=|  mask(MainDlg_basic_Code){SampleTime=-1, ttlib=IO_Blk_Lib_TTC500, ttDescription=MainDlg_basic, tt_iolib_version=0.25, baudrate_CAN0=baudrate_CAN0, tseg1_CAN0=tseg1_CAN0, tseg2_CAN0=tseg2_CAN0, sjw_CAN0=sjw_CAN0, brp_CAN0=brp_CAN0, baudrate_CAN1=baudrate_CAN1, tseg1_CAN1=tseg1_CAN1, tseg2_CAN1=tseg2_CAN1, sjw_CAN1=sjw_CAN1, brp_CAN1=brp_CAN1, baudrate_CAN2=baudrate_CAN2, tseg1_CAN2=tseg1_CAN2, tseg2_CAN2=tseg2_CAN2, sjw_CAN2=sjw_CAN2, brp_CAN2=brp_CAN2, baudrate_CAN3=baudrate_CAN3, baudrate_CAN4=baudrate_CAN4, baudrate_CAN5=baudrate_CAN5, baudrate_CAN6=baudrate_CAN6, tseg1=tseg1, tseg2=tseg2, sjw=sjw, Duration_ms=Duration_ms, glitch_filter_time=glitch_filter_time, watchdog_window_size=watchdog_window_size, watchdog_reset_behavior=watchdog_reset_behavior, brp=brp, Major_Number=Major_Number, Minor_Number=Minor_Number, Revison_Number=Revison_Number, Node_Number=Node_Number, Enable_Reset_by_TTCDownloader=Enable_Reset_by_TTCDownloader, Enable_CCP=Enable_CCP, CRO_ID=CRO_ID, DTO_ID=DTO_ID, CCP_Station_Addr=CCP_Station_Addr, CCP_Station_ID=CCP_Station_ID, CPP_channel=CPP_channel, CPP_id_format=CPP_id_format, bEnable_DAQ0=bEnable_DAQ0, bEnable_DAQ1_2=bEnable_DAQ1_2, ODT_total=ODT_total, bEnable_ErrorCBAction=bEnable_ErrorCBAction, bDIAG_ERR_DISABLE_SSW0=bDIAG_ERR_DISABLE_SSW0, bDIAG_ERR_DISABLE_SSW1=bDIAG_ERR_DISABLE_SSW1, bDIAG_ERR_DISABLE_SSW2=bDIAG_ERR_DISABLE_SSW2, bFlashOverEthernet=bFlashOverEthernet}
      | try
      | %
      | %Upgrade Information - standard BEGIN
      | new_color = 'blue';
      | new_ver = '0.25';
      | act_ver = get_param(gcb,'tt_iolib_version');
      | if not(strcmp(act_ver,new_ver))
      |     disp(['Upgrade block: ',gcb,char(10),'       Version: ',act_ver,' to ',new_ver]);
      |     %switch - case for specific upgrade information e.g. additional parameter required 
      |     %Change appearance and version information
      |     set_param(gcb,'ForegroundColor',new_color);
      |     set_param(gcb,'tt_iolib_version',new_ver);
      | end
      | %Upgrade Information - standard END
      | catch
      | %Standard catch section BEGIN
      | errordlg('An error occurred in a callback of the TTC580-BlockLib. Please open the Diagnostic Viewer for further details');
      | disp(' ');
      | disp('------------------------------------------------------------');
      | disp('An error occurred in a callback of the TTC580-BlockLib.');
      | disp(['Please check the parameters in the mask of ',gcb]);
      | disp('If you do not encounter any violations, then please '); 
      | disp('copy the following lines and report this to support@ttcontrol.com ');
      | disp('<< begin of error message dump >>');
      | disp(['Version of TTC580-BlockLib: ', get_param(gcb,'tt_iolib_version')]);
      | disp(get_param(gcb,'ttDescription'));
      | disp(gcb);
      | x=lasterror;disp(x.message);
      | disp(get_param(gcb,'MaskValues'));
      | disp(version);
      | disp(computer);
      | disp('<< end of error message dump >>');
      | disp('------------------------------------------------------------');
      | disp(' ');
      | %Standard catch section END
      | end
      mask help:
      | Block representing the handler for main environment-settings of the applications to be run on a TTC580.
      | Generation of <model>_main.c
      mask init:
      | %
      settings: CopyFcn=%deleted
      mask Help: No further help available for this block
      mask Callback baudrate_CAN0: %
      mask Callback tseg1_CAN0: %
      mask Callback tseg2_CAN0: %
      mask Callback sjw_CAN0: %
      mask Callback brp_CAN0: %
      mask Callback baudrate_CAN1: %
      mask Callback tseg1_CAN1: %
      mask Callback tseg2_CAN1: %
      mask Callback sjw_CAN1: %
      mask Callback brp_CAN1: %
      mask Callback baudrate_CAN2: %
      mask Callback tseg1_CAN2: %
      mask Callback tseg2_CAN2: %
      mask Callback sjw_CAN2: %
      mask Callback brp_CAN2: %
      mask Callback baudrate_CAN3: %
      mask Callback baudrate_CAN4: %
      mask Callback baudrate_CAN5: %
      mask Callback baudrate_CAN6: %
      mask Callback tseg1: %
      mask Callback tseg2: %
      mask Callback sjw: %
      mask Callback Duration_ms: %
      mask Callback glitch_filter_time: %
      mask Callback watchdog_window_size: %
      mask Callback watchdog_reset_behavior: %
      mask Callback brp: %
      mask Callback Major_Number: %
      mask Callback Minor_Number: %
      mask Callback Revison_Number: %
      mask Callback Node_Number: %
      mask Callback Enable_Reset_by_TTCDownloader: %
      mask Callback Enable_CCP: %
      mask Callback CRO_ID: %
      mask Callback DTO_ID: %
      mask Callback CCP_Station_Addr: %
      mask Callback CCP_Station_ID: %
      mask Callback CPP_channel: %
      mask Callback CPP_id_format: %
      mask Callback bEnable_DAQ0: %
      mask Callback bEnable_DAQ1_2: %
      mask Callback ODT_total: %
      mask Callback bEnable_ErrorCBAction: %
      mask Callback bDIAG_ERR_DISABLE_SSW0: %
      mask Callback bDIAG_ERR_DISABLE_SSW1: %
      mask Callback bDIAG_ERR_DISABLE_SSW2: %
      mask Callback bFlashOverEthernet:
      | try
      | s_ParameterDecision = 'bFlashOverEthernet'; %Deside on this parameter
      | c_ValuesDecision={'on'}; %Positive DescitionValues
      | s_ParameterInvisible = 'Enable_Reset_by_TTCDownloader'; %Make this invisible
      | %trim
      | if ischar(s_ParameterInvisible)%if secttion for compatibility reasons of template
      |     cs_ParameterInvisible = {s_ParameterInvisible};
      | else
      |     cs_ParameterInvisible = s_ParameterInvisible;
      | end
      | s_ParameterDecision = strtrim(s_ParameterDecision);
      | c_ValuesDecision = strtrim(c_ValuesDecision);
      | for j=1:length(cs_ParameterInvisible)
      |   s_ParameterInvisible = strtrim(cs_ParameterInvisible{j});
      |   c_MaskVisibilities=get_param(gcb,'MaskVisibilities');
      |   %check consistency
      |   idx=strmatch(s_ParameterInvisible,get_param(gcb,'MaskNames'),'exact');
      |   c_MaskVisibilities{idx}='on'; %default
      |     for i = 1: length(c_ValuesDecision)
      |         if ~isempty(strmatch(get_param(gcb, s_ParameterDecision), c_ValuesDecision{i},'exact'))
      |            c_MaskVisibilities{idx}='off';
      |         end
      |     end
      |   set_param(gcb,'MaskVisibilities',c_MaskVisibilities);
      | end
      | catch
      | %Standard catch section BEGIN
      | errordlg('An error occurred in a callback of the TTC580-BlockLib. Please open the Diagnostic Viewer for further details');
      | disp(' ');
      | disp('------------------------------------------------------------');
      | disp('An error occurred in a callback of the TTC580-BlockLib.');
      | disp(['Please check the parameters in the mask of ',gcb]);
      | disp('If you do not encounter any violations, then please ');
      | disp('copy the following lines and report this to support@ttcontrol.com ');
      | disp('<< begin of error message dump >>');
      | disp(['Version of TTC580-BlockLib: ', get_param(gcb,'tt_iolib_version')]);
      | disp(get_param(gcb,'ttDescription'));
      | disp(gcb);
      | x=lasterror;disp(x.message);
      | disp(get_param(gcb,'MaskValues'));
      | disp(version);
      | disp(computer);
      | disp('<< end of error message dump >>');
      | disp('------------------------------------------------------------');
      | disp(' ');
      | %Standard catch section END
      | end
  ErrorCode : Outport  VectorParamsAs1DForOutWhenUnconnected=off
  ExecutionTime : Outport  Port=2  VectorParamsAs1DForOutWhenUnconnected=off
  wires:
  MainDlg_basic/2(ExecutionTime) -> ExecutionTime/1
  MainDlg_basic/1(ErrorCode) -> ErrorCode/1

== system IOBlock_Library_TTC580/System  Blocks TTC580 IOlib/Postrun_Enable ==
  enable : Inport  OutDataTypeStr=boolean  PortDimensions=1
  Compare To Zero : simulink/Logic and Bit Operations/Compare To Zero  relop=~=  OutDataTypeStr=boolean  ZeroCross=off
  Data Type Conversion : DataTypeConversion  OutDataTypeStr=uint8
  IO_POWER_Get_KL15 : Subsystem  LoadFcn=|  mask(IO_POWER_Get_Code){SampleTime=-1, ttlib=IO_Blk_Lib_TTC500, ttDescription=IO_POWER_Get, tt_iolib_version=0.19, pin=IO_K15}
      | try
      | %
      | %Upgrade Information - standard BEGIN
      | new_color = 'blue';
      | new_ver = '0.19';
      | act_ver = get_param(gcb,'tt_iolib_version');
      | if not(strcmp(act_ver,new_ver))
      |     disp(['Upgrade block: ',gcb,char(10),'       Version: ',act_ver,' -> ',new_ver]);
      |     %switch - case for specific upgrade information e.g. additional parameter required 
      |     %Change appearance and version information
      |     set_param(gcb,'ForegroundColor',new_color);
      |     set_param(gcb,'tt_iolib_version',new_ver);
      | end
      | %Upgrade Information - standard END
      | catch
      | %Standard catch section BEGIN 
      | disp(' ');
      | disp('------------------------------------------------------------');
      | disp('An error occurred in a callback of the TTC580-BlockLib.');
      | disp(['Please check the parameters in the mask of ',gcb]);
      | disp('If you do not encounter any violations, then please '); 
      | disp('copy the following lines and report this to support@ttcontrol.com ');
      | disp('<< begin of error message dump >>');
      | disp(['Version of TTC580-BlockLib: ', get_param(gcb,'tt_iolib_version')]);
      | disp(get_param(gcb,'ttDescription'));
      | disp(gcb);
      | x=lasterror;disp(x.message);
      | disp(get_param(gcb,'MaskValues'));
      | disp(version);
      | disp(computer);
      | disp('<< end of error message dump >>');
      | disp('------------------------------------------------------------');
      | disp(' ');
      | %Standard catch section END
      | end
      mask help: Returns the current state of a POWER feature.
      mask init:
      | %
      settings: CopyFcn=%deleted
      mask Help: web(which('IO_POWER.h'))
      mask TypeOptions pin: IO_INT_POWERSTAGE_ENABLE | IO_SENSOR_SUPPLY_0 | IO_SENSOR_SUPPLY_1 | IO_SENSOR_SUPPLY_2 | IO_INT_SAFETY_SW_0 | IO_INT_SAFETY_SW_1 | IO_INT_SAFETY_SW_2 | IO_K15 | IO_WAKEUP
      mask Callback pin: %
  IO_POWER_Set_KL15 : Subsystem  LoadFcn=|  mask(IO_POWER_Set_Code){SampleTime=-1, ttlib=IO_Blk_Lib_TTC500, ttDescription=IO_POWER_Set, tt_iolib_version=0.19, pin=IO_K15}
      | try
      | %
      | %Upgrade Information - standard BEGIN
      | new_color = 'blue';
      | new_ver = '0.19';
      | act_ver = get_param(gcb,'tt_iolib_version');
      | if not(strcmp(act_ver,new_ver))
      |     disp(['Upgrade block: ',gcb,char(10),'       Version: ',act_ver,' -> ',new_ver]);
      |     %switch - case for specific upgrade information e.g. additional parameter required 
      |     %Change appearance and version information
      |     set_param(gcb,'ForegroundColor',new_color);
      |     set_param(gcb,'tt_iolib_version',new_ver);
      | end
      | %Upgrade Information - standard END
      | catch
      | %Standard catch section BEGIN 
      | disp(' ');
      | disp('------------------------------------------------------------');
      | disp('An error occurred in a callback of the TTC580-BlockLib.');
      | disp(['Please check the parameters in the mask of ',gcb]);
      | disp('If you do not encounter any violations, then please '); 
      | disp('copy the following lines and report this to support@ttcontrol.com ');
      | disp('<< begin of error message dump >>');
      | disp(['Version of TTC580-BlockLib: ', get_param(gcb,'tt_iolib_version')]);
      | disp(get_param(gcb,'ttDescription'));
      | disp(gcb);
      | x=lasterror;disp(x.message);
      | disp(get_param(gcb,'MaskValues'));
      | disp(version);
      | disp(computer);
      | disp('<< end of error message dump >>');
      | disp('------------------------------------------------------------');
      | disp(' ');
      | %Standard catch section END
      | end
      mask help: Sets a certain mode of the Power IC.
      mask init:
      | %
      settings: CopyFcn=%deleted
      mask Help: web(which('IO_POWER.h'))
      mask TypeOptions pin: IO_INT_POWERSTAGE_ENABLE | IO_SENSOR_SUPPLY_0 | IO_SENSOR_SUPPLY_1 | IO_SENSOR_SUPPLY_2 | IO_INT_SAFETY_SW_0 | IO_INT_SAFETY_SW_1 | IO_INT_SAFETY_SW_2 | IO_K15 | IO_WAKEUP
      mask Callback pin: %
  Logical Operator : Logic  Operator=OR  AllPortsSameDT=off  OutDataTypeStr=boolean
  Terminator_enable : Terminator
  Terminator_enable1 : Terminator
  wires:
  IO_POWER_Set_KL15/1(ErrorCode) -> Terminator_enable/1
  Data Type Conversion/1 -> IO_POWER_Set_KL15/1(mode)
  IO_POWER_Get_KL15/1(ErrorCode) -> Terminator_enable1/1
  IO_POWER_Get_KL15/2(state) -> Compare To Zero/1
  enable/1 -> Logical Operator/2
  Logical Operator/1 -> Data Type Conversion/1
  Compare To Zero/1 -> Logical Operator/1
